simulink subsystem "MCD"  (R2023b)
settings: Solver=VariableStepAuto  StartTime=0.0  StopTime=10.0  RelTol=1e-3
settings Model: Creator=Diego  LastModifiedBy=Diego

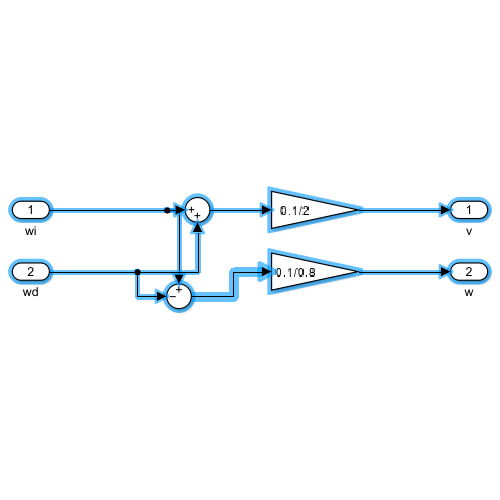
[thumbnail: Simulink's stored preview of the top-level diagram]
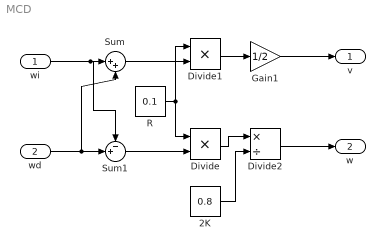
== system MCD ==
  wi : Inport
  wd : Inport  Port=2
  2K : Constant  Value=0.8
  Divide : Product
  Divide1 : Product
  Divide2 : Product  Inputs=*/
  Gain1 : Gain  Gain=1/2
  R : Constant  Value=0.1
  Sum : Sum  Inputs=|++
  Sum1 : Sum  Inputs=-+|
  v : Outport
  w : Outport  Port=2
  wires:
  Divide2/1 -> w/1
  Gain1/1 -> v/1
  wi/1 -> Sum1/1, Sum/1
  wd/1 -> Sum1/2, Sum/2
  Divide1/1 -> Gain1/1
  Sum/1 -> Divide1/2
  R/1 -> Divide/1, Divide1/1
  Sum1/1 -> Divide/2
  2K/1 -> Divide2/2
  Divide/1 -> Divide2/1
